simulink model "Landing_VV"  (R2018b)
settings: Solver=ode4  StartTime=0.0  StopTime=simTime  FixedStep=dt  RelTol=1e-3
InitFcn:
  | SimulationInitialization
StopFcn:
  | SimulationEnd
values from neighbouring files (symbols this model uses):
  Alt = 1000 + TerrainHeight    [SimulationStateConfig.m]
  C = GeneticOpt.C    [SimulationCostFunction.m]
  CartRange_m = MaxAftCartLocX_m - MaxFwdCartLocX_m    (= 1.8505)    [SimulationWSMConfig.m]
  DP_init = 0.5*1.225*V_init^2    [SimulationControlConfig16P.m]    (also in SimulationControlConfig16P_F0.m; SimulationControlConfig16P_F2.m; SimulationControlConfig16P_LEGACY.m; SimulationControlConfigTAILLESS.m)
  dt = DLLSim.dt    [SimulationTimeStep.m]    (also in SimulationTrim.m = 0.02)
  ElevatorMax = 25    [SimulationControlConfig16P.m]    (also in SimulationControlConfig16P_F0.m; SimulationControlConfig16P_F2.m; SimulationControlConfig16P_LEGACY.m; SimulationControlConfigTAILLESS.m)
  EngineLhFuelCut = 0    [SimulationAircraftConfig.m]
  EngineRhFuelCut = 0    [SimulationAircraftConfig.m]
  ftvStaticPositionError = 1/1.18    (= 0.847457627119)    [SimulationSensorConfig16P.m]    (also in SimulationSensorConfig16P_LEGACY.m; SimulationSensorConfigTAILLESS7P.m = 1; SimulationSensorConfigUTAIL7P.m = 1)
  g = 9.81    [SimulationStateConfig.m]
  GustSpd_Kts = testPlans(testIndx).gustSpd    [SimulationStateConfig.m]
  GustTriggerVal = testPlans(testIndx).gustTriggerVal    [SimulationStateConfig.m]
  m = 13.1784    [InertiaEstimatorBWB.m]    (also in SimulationControlConfig16P.m = MassBWB; SimulationControlConfig16P_F0.m = MassBWB; SimulationControlConfig16P_F2.m = MassBWB; SimulationControlConfig16P_LEGACY.m = MassBWB)
  MaxAftCartLocX_m = 2.5327    [SimulationWSMConfig.m]
  MaxFwdCartLocX_m = 0.6822    [SimulationWSMConfig.m]
  nMax_User = 2.6    [SimulationControlConfig16P.m]    (also in SimulationControlConfig16P_F0.m; SimulationControlConfig16P_F2.m; SimulationControlConfig16P_LEGACY.m; SimulationControlConfigTAILLESS.m = 2.5)
  nMin_User = -1.3    [SimulationControlConfig16P.m]    (also in SimulationControlConfig16P_F0.m; SimulationControlConfig16P_F2.m; SimulationControlConfig16P_LEGACY.m; SimulationControlConfigTAILLESS.m = -1)
  SimObj = CompiledSimulink(DLL_Name)    [SimulationTrim.m]
  taxiTrackOffset = testPlans(testIndx).rolloutTrackOffset    [SimulationControlConfig16P.m]    (also in SimulationControlConfig16P_F0.m; SimulationControlConfig16P_F2.m; SimulationControlConfig16P_LEGACY.m; SimulationControlConfigTAILLESS.m)
  V_init = Speed*0.5144    [SimulationControlConfig16P.m]    (also in SimulationControlConfig16P_F0.m; SimulationControlConfig16P_F2.m; SimulationControlConfig16P_LEGACY.m; SimulationControlConfigTAILLESS.m)
  WindDir_Deg = testPlans(testIndx).winds(3)    [SimulationStateConfig.m]
  WindSpd_Kts = testPlans(testIndx).winds(1)    [SimulationStateConfig.m]
  WindVertSpd_Kts = 0    [SimulationStateConfig.m]
  WOWarmed = 1    [SimulationControlConfig16P.m]    (also in SimulationControlConfig16P_F0.m; SimulationControlConfig16P_F2.m; SimulationControlConfig16P_LEGACY.m; SimulationControlConfigTAILLESS.m)
undefined symbols (not defined in the file or in its folder): DiscIntNeverNeededParam, DLLSim, DLLSimStep, sigbuilder_block, Trim_piccoloInCmd, Trim_REFSI_FD_IN_nmodeCgShifterCmd_Flag, Trim_REFSI_FD_IN_nmodeCgShifterCmd_Ft, Trim_REFSI_FD_IN_nmodeCgShifterNRCActive, WSMCart
libraries: Lib_Piccolo x16, simulink x10, aerolibatmos2 x2, Lib_HStab x1
(part 1 of 3)
settings Model: Creator=JSheng  LastModifiedBy=JCdFFigueira

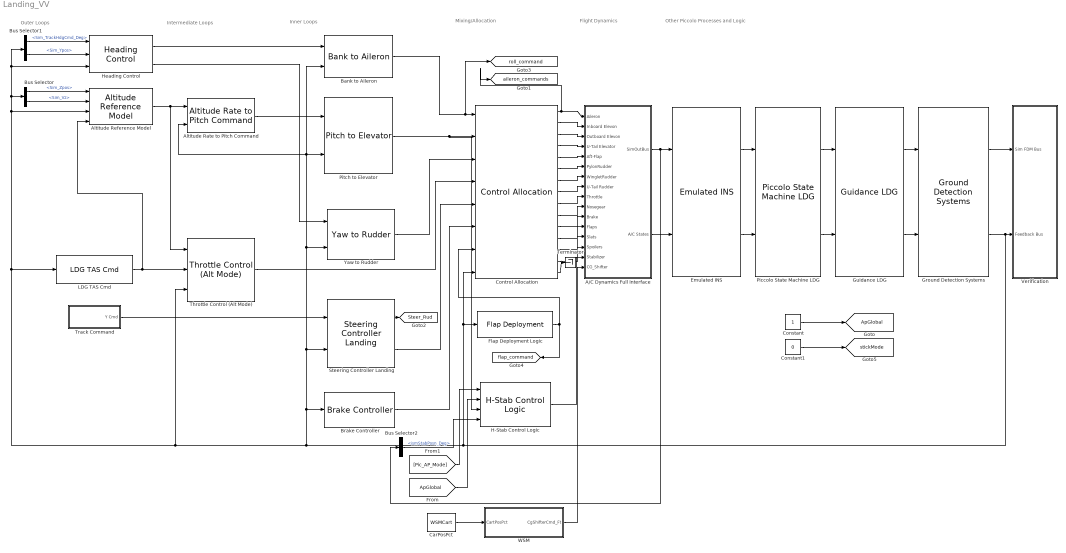
== system Landing_VV ==
  note: Outer Loops
  note: Intermediate Loops
  note: Inner Loops
  note: Flight Dynamics
  note: Other Piccolo Processes and Logic
  note: Mixing/Allocation
  A/C Dynamics Full Interface : Subsystem  AncestorBlock=Lib_Piccolo/A//C Dynamics Full Interface
  Altitude Rate to Pitch Command : Lib_Piccolo/Altitude Rate to Pitch Command  SystemSampleTime=-1
  Altitude Reference Model : Lib_Piccolo/Altitude Reference Model  SystemSampleTime=-1
  Bank to Aileron : Lib_Piccolo/Bank to Aileron  SystemSampleTime=-1
  Brake Controller : Lib_Piccolo/Brake Controller  SystemSampleTime=-1
  Bus Selector : BusSelector  OutputSignals=Sim_Zpos,Sim_Vz
  Bus Selector1 : BusSelector  OutputSignals=Sim_TrackHdgCmd_Deg,Sim_Ypos
  Bus Selector2 : BusSelector  OutputSignals=ismStabPosn_Deg
  CarPosPct : Constant  Value=WSMCart
  Constant : Constant
  Constant1 : Constant  Value=0
  Control Allocation : Lib_Piccolo/Control Allocation  SystemSampleTime=-1
  Emulated INS : Lib_Piccolo/Emulated INS  SystemSampleTime=-1
  Flap Deployment Logic : Lib_Piccolo/Flap Deployment  SystemSampleTime=-1
  Ground Detection Systems : Lib_Piccolo/Ground Detection Systems  SystemSampleTime=-1
  Guidance LDG : Lib_Piccolo/Guidance LDG  SystemSampleTime=-1
  H-Stab Control Logic : Lib_HStab/H-Stab Control Logic  SystemSampleTime=-1  VariantControl=Variant1  LabelModeActiveChoice=FTV == 4
  Heading Control : Lib_Piccolo/Heading Control  SystemSampleTime=-1
  LDG TAS Cmd : Lib_Piccolo/LDG TAS Cmd  SystemSampleTime=-1
  Piccolo State Machine LDG : Lib_Piccolo/Piccolo State Machine LDG  SystemSampleTime=-1
  Pitch to Elevator : Lib_Piccolo/Pitch to Elevator  SystemSampleTime=-1
  Steering Controller Landing : Lib_Piccolo/Steering Controller Landing  SystemSampleTime=-1
  Terminator : Terminator
  Throttle Control (Alt Mode) : Lib_Piccolo/Throttle Control (Alt Mode)  SystemSampleTime=-1
  Track Command : Subsystem
  Verification : Subsystem
  WSM : Subsystem
  Yaw to Rudder : Lib_Piccolo/Yaw to Rudder  SystemSampleTime=-1
  tag scope: ApGlobal=global, Steer_Rud=global, aileron_commands=global, flap_command=global, roll_command=global, stickMode=global
  wires:
  Pitch to Elevator/1 -> H-Stab Control Logic/3, Control Allocation/2
  Altitude Rate to Pitch Command/1 -> Pitch to Elevator/1
  Bank to Aileron/1 -> [roll_command], Control Allocation/1
  Control Allocation/1 -> [aileron_commands], A/C Dynamics Full Interface/1(Aileron)
  Control Allocation/2 -> A/C Dynamics Full Interface/2(Inboard Elevon)
  Control Allocation/3 -> A/C Dynamics Full Interface/3(Outboard Elevon)
  Control Allocation/4 -> A/C Dynamics Full Interface/4(U-Tail Elevator)
  Control Allocation/5 -> A/C Dynamics Full Interface/5(Aft-Flap)
  Control Allocation/6 -> A/C Dynamics Full Interface/6("PylonRudder ")
  Control Allocation/7 -> A/C Dynamics Full Interface/7(WingletRudder)
  Control Allocation/8 -> A/C Dynamics Full Interface/8(U-Tail Rudder)
  Control Allocation/9 -> A/C Dynamics Full Interface/9("Throttle ")
  Throttle Control (Alt Mode)/1 -> Control Allocation/4
  Heading Control/1 -> Bank to Aileron/1
  A/C Dynamics Full Interface/2(A/C States) -> Emulated INS/2
  LDG TAS Cmd/1 -> Throttle Control (Alt Mode)/2, Altitude Reference Model/4
  A/C Dynamics Full Interface/1(SimOutBus) -> Bus Selector2/1, Emulated INS/1
  Control Allocation/10 -> A/C Dynamics Full Interface/10(Nosegear)
  Control Allocation/11 -> A/C Dynamics Full Interface/11(Brake)
  Track Command/1(Y Cmd) -> Steering Controller Landing/1
  Brake Controller/1 -> Control Allocation/6
  Steering Controller Landing/2 -> Control Allocation/5
  Steering Controller Landing/1 -> [Steer_Rud]
  Yaw to Rudder/1 -> Control Allocation/3
  Emulated INS/2 -> Piccolo State Machine LDG/2
  Emulated INS/1 -> Piccolo State Machine LDG/1
  Ground Detection Systems/2 -> Verification/2(Feedback Bus), LDG TAS Cmd/1, Bus Selector/1, Heading Control/3, Bus Selector1/1, Altitude Reference Model/3, Throttle Control (Alt Mode)/3, Brake Controller/1, Steering Controller Landing/2, Pitch to Elevator/2, Bank to Aileron/2, Altitude Rate to Pitch Command/2, Yaw to Rudder/2, Flap Deployment Logic/1, Control Allocation/8
  Ground Detection Systems/1 -> Verification/1(Sim FDM Bus)
  Piccolo State Machine LDG/2 -> Guidance LDG/2
  Guidance LDG/2 -> Ground Detection Systems/2
  Piccolo State Machine LDG/1 -> Guidance LDG/1
  Guidance LDG/1 -> Ground Detection Systems/1
  Altitude Reference Model/1 -> Throttle Control (Alt Mode)/1, Altitude Rate to Pitch Command/1
  Bus Selector/2 -> Altitude Reference Model/2  "<Sim_Vz>"
  Bus Selector/1 -> Altitude Reference Model/1  "<Sim_Zpos>"
  Bus Selector1/2 -> Heading Control/2  "<Sim_Ypos>"
  Heading Control/2 -> Yaw to Rudder/1
  Bus Selector1/1 -> Heading Control/1  "<Sim_TrackHdgCmd_Deg>"
  Control Allocation/12 -> A/C Dynamics Full Interface/12(Flaps)
  Control Allocation/13 -> A/C Dynamics Full Interface/13(Slats)
  Control Allocation/14 -> A/C Dynamics Full Interface/14(Spoilers)
  Constant/1 -> [ApGlobal]
  Control Allocation/15 -> Terminator/1
  Flap Deployment Logic/1 -> [flap_command], Control Allocation/7
  Constant1/1 -> [stickMode]
  H-Stab Control Logic/1 -> A/C Dynamics Full Interface/15(Stabilizer)
  [ApGlobal] -> H-Stab Control Logic/2
  [Pic_AP_Mode] -> H-Stab Control Logic/1
  Bus Selector2/1 -> H-Stab Control Logic/4  "<ismStabPosn_Deg>"
  WSM/1(CgShifterCmd_Ft) -> A/C Dynamics Full Interface/16(CG_Shifter)
  CarPosPct/1 -> WSM/1(CartPosPct)

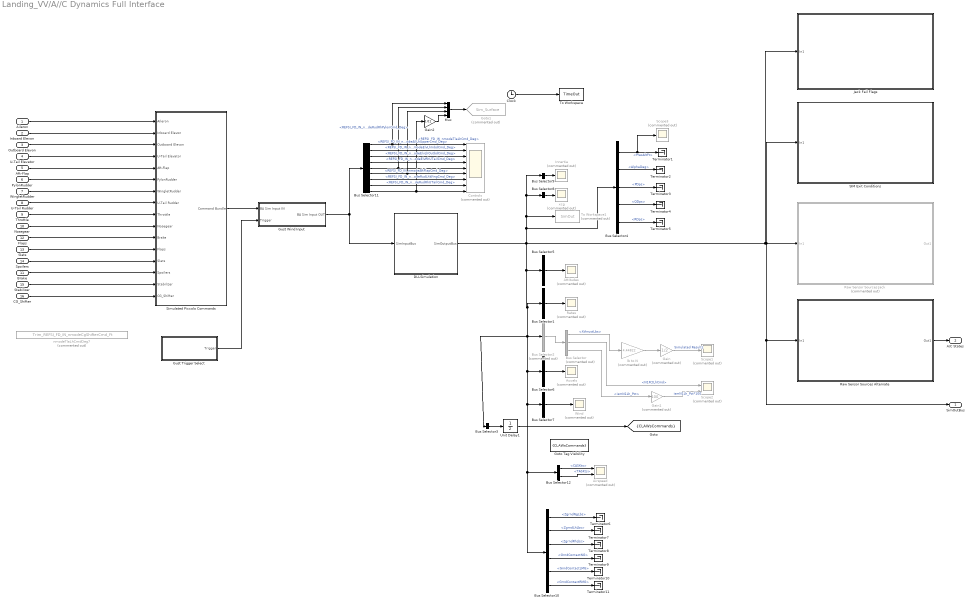
== system Landing_VV/A//C Dynamics Full Interface ==
  Aileron : Inport
  Inboard Elevon : Inport  Port=2
  Outboard Elevon : Inport  Port=3
  U-Tail Elevator : Inport  Port=4
  Aft-Flap : Inport  Port=5
  "PylonRudder " : Inport  Port=6
  WingletRudder : Inport  Port=7
  U-Tail Rudder : Inport  Port=8
  "Throttle " : Inport  Port=9
  Nosegear : Inport  Port=10
  Brake : Inport  Port=11
  Flaps : Inport  Port=12
  Slats : Inport  Port=13
  Spoilers : Inport  Port=14
  Stabilizer : Inport  Port=15
  CG_Shifter : Inport  Port=16
  Accels : Scope  Commented=on
  Airspeed : Scope  Commented=on  NumInputPorts=2
  Attitudes : Scope  Commented=on
  Bus Selector : BusSelector  Commented=on  OutputSignals=XthrustLbs,N1PctLhCmd,ismN1Lh_Pct
  Bus Selector1 : BusSelector  OutputSignals=PDps,QDps,RDps  OutputAsBus=on
  Bus Selector10 : BusSelector  OutputSignals=ZgrndNgLbs,ZgrndLhLbs,ZgrndRhLbs,GrndContactNG,GrndContactLMG,GrndContactRMG
  Bus Selector11 : BusSelector  OutputSignals=REFSI_FD_IN_nmodeAilLhUpperCmd_Deg,REFSI_FD_IN_nmodeElvLhInbdCmd_Deg,REFSI_FD_IN_nmodeElvLhOutbdCmd_Deg,REFSI_FD_IN_nmodeElvRhUTailCmd_Deg,REFSI_FD_IN_nmodeAftFlapCmd_Deg,REFSI_FD_IN_nmodeRudRhPylonCmd_Deg,REFSI_FD_IN_nmodeRudLhWingCmd_Deg,REFSI_FD_IN_nmodeRudRhUTailCmd_Deg,REFSI_FD_IN_nmodeTlaLhCmd_Deg
  Bus Selector12 : BusSelector  OutputSignals=CASKts,TASKts
  Bus Selector2 : BusSelector  Commented=on  OutputSignals=XthrustLbs,N1PctLhCmd,ismN1Lh_Pct,ismFuelBurnRateLh_Lpm,ismFuelBurntLh_Lbs  OutputAsBus=on
  Bus Selector3 : BusSelector  OutputSignals=REFSI_AC_OUT_nmodeRudLhWingCmd_Deg,REFSI_AC_OUT_nmodeAilLhLowerCmd_Deg,REFSI_AC_OUT_nmodeAilLhUpperCmd_Deg,REFSI_AC_OUT_nmodeElvLhOutbdCmd_Deg,REFSI_AC_OUT_nmodeElvLhInbdCmd_Deg,REFSI_AC_OUT_nmodeRudLhPylonCmd_Deg,REFSI_AC_OUT_nmodeRudLhUTailCmd_Deg,REFSI_AC_OUT_nmodeElvLhUTailCmd_Deg,REFSI_AC_OUT_nmodeAftFlapCmd_Deg,REFSI_AC_OUT_nmodeElvRhUTailCmd_Deg,REFSI_AC_OUT_nmodeRudRhUTailCmd_Deg,REFSI_AC_OUT_nmodeRudRhPylonCmd_Deg,REFSI_AC_OUT_nmodeElvRhInbdCmd_Deg,REFSI_AC_OUT_nmodeElvRhOutbdCmd_Deg,REFSI_AC_OUT_nmodeAilRhUpperCmd_Deg,REFSI_AC_OUT_nmodeAilRhLowerCmd_Deg,REFSI_AC_OUT_nmodeRudRhWingCmd_Deg  OutputAsBus=on
  Bus Selector4 : BusSelector  OutputSignals=PresAltFt,AlphaDeg,PDps,QDps,RDps
  Bus Selector5 : BusSelector  OutputSignals=PhiDeg,ThetaDeg,PsiDeg  OutputAsBus=on
  Bus Selector6 : BusSelector  OutputSignals=NxG,NyG,NzG  OutputAsBus=on
  Bus Selector7 : BusSelector  OutputSignals=WindUFtps,WindVFtps,WindWFtps  OutputAsBus=on
  Bus Selector8 : BusSelector  OutputSignals=XcgPctMAC  OutputAsBus=on
  Bus Selector9 : BusSelector  OutputSignals=IxxLbsInch2,IyyLbsInch2,IzzLbsInch2,IxzLbsInch2  OutputAsBus=on
  Clock : Clock
  Controls : Scope  Commented=on  NumInputPorts=9
  DLLSimulation : Subsystem
  Gain : Gain  Commented=on  Gain=1/2
  Gain1 : Gain  Commented=on  Gain=100
  Gain2 : Gain  Gain=0.01
  Goto Tag Visibility : GotoTagVisibility  GotoTag=CLAWsCommands
  Goto1 : Goto  Commented=on  GotoTag=Sim_Surface  TagVisibility=global
  Gust Trigger Select : Subsystem  Variant=on
  Gust Wind Input : Subsystem  Variant=on
  Innertia : Scope  Commented=on
  Jack Fail Flags : Subsystem
  Mux : Mux
  Rates : Scope  Commented=on
  Raw Sensor Sources Alternate : Subsystem
  Raw Sensor Sources Jack : Subsystem  Commented=on
  SIM Exit Conditions : Subsystem
  Scope1 : Scope  Commented=on
  Scope2 : Scope  Commented=on  NumInputPorts=2
  Scope3 : Scope  Commented=on
  Simulated Piccolo Commands : Subsystem  Variant=on
  Terminator{1..11} (11 alike) : Terminator
  To Workspace : ToWorkspace  VariableName=TimeOut  SaveFormat=Structure With Time  SampleTime=-1
  To Workspace1 : ToWorkspace  Commented=on  VariableName=SimOut  SaveFormat=Timeseries  SampleTime=-1
  Unit Delay1 : UnitDelay  SampleTime=-1
  Wind : Scope  Commented=on
  lb to N : Gain  Commented=on  Gain=4.44822
  nmodeTlaLhCmdDeg7 : Constant  Commented=on  Value=Trim_REFSI_FD_IN_nmodeCgShifterCmd_Ft
  xcg : Scope  Commented=on
  SimOutBus : Outport
  A/C States : Outport  Port=2
  tag scope: CLAWsCommands=scoped
  wires:
  "Throttle "/1 -> Simulated Piccolo Commands/9("Throttle ")
  Outboard Elevon/1 -> Simulated Piccolo Commands/3(Outboard Elevon)
  Nosegear/1 -> Simulated Piccolo Commands/10(Nosegear)
  Spoilers/1 -> Simulated Piccolo Commands/13(Slats)
  Gust Trigger Select/1(Trigger) -> Gust Wind Input/2(Trigger)
  Slats/1 -> Simulated Piccolo Commands/12(Flaps)
  Flaps/1 -> Simulated Piccolo Commands/11(Brake)
  Stabilizer/1 -> Simulated Piccolo Commands/15(Stabilizer)
  Inboard Elevon/1 -> Simulated Piccolo Commands/2(Inboard Elevon)
  U-Tail Elevator/1 -> Simulated Piccolo Commands/4(U-Tail Elevator)
  U-Tail Rudder/1 -> Simulated Piccolo Commands/8(U-Tail Rudder)
  Simulated Piccolo Commands/1(Command Bundle) -> Gust Wind Input/1(BA Sim Input IN)
  "PylonRudder "/1 -> Simulated Piccolo Commands/6("PylonRudder ")
  Brake/1 -> Simulated Piccolo Commands/14(Spoilers)
  WingletRudder/1 -> Simulated Piccolo Commands/7(WingletRudder)
  Aft-Flap/1 -> Simulated Piccolo Commands/5(Aft-Flap)
  Aileron/1 -> Simulated Piccolo Commands/1(Aileron)
  Raw Sensor Sources Alternate/1(Out1) -> A/C States/1
  DLLSimulation/1(SimOutputBus) -> To Workspace1/1, Bus Selector8/1, Bus Selector9/1, Bus Selector4/1, Bus Selector1/1, Bus Selector2/1, Bus Selector3/1, Bus Selector6/1, Bus Selector7/1, Bus Selector12/1, Bus Selector10/1, Bus Selector5/1, Raw Sensor Sources Jack/1(In1), SimOutBus/1, Raw Sensor Sources Alternate/1(In1), SIM Exit Conditions/1(In1), Jack Fail Flags/1(In1)
  Bus Selector10/6 -> Terminator11/1  "<GrndContactRMG>"
  Bus Selector10/5 -> Terminator10/1  "<GrndContactLMG>"
  Bus Selector10/4 -> Terminator9/1  "<GrndContactNG>"
  Bus Selector10/3 -> Terminator8/1  "<ZgrndRhLbs>"
  Bus Selector10/2 -> Terminator7/1  "<ZgrndLhLbs>"
  Bus Selector10/1 -> Terminator6/1  "<ZgrndNgLbs>"
  Gain2/1 -> Mux/4
  Mux/1 -> Goto1/1
  Bus Selector11/9 -> Controls/9, Gain2/1  "<REFSI_FD_IN_nmodeTlaLhCmd_Deg>"
  Bus Selector11/8 -> Controls/8  "<REFSI_FD_IN_nmodeRudRhUTailCmd_Deg>"
  Bus Selector11/7 -> Controls/7  "<REFSI_FD_IN_nmodeRudLhWingCmd_Deg>"
  Bus Selector11/6 -> Mux/3, Controls/6  "<REFSI_FD_IN_nmodeRudRhPylonCmd_Deg>"
  Bus Selector11/5 -> Mux/2, Controls/5  "<REFSI_FD_IN_nmodeAftFlapCmd_Deg>"
  Bus Selector11/4 -> Controls/4  "<REFSI_FD_IN_nmodeElvRhUTailCmd_Deg>"
  Bus Selector11/3 -> Controls/3  "<REFSI_FD_IN_nmodeElvLhOutbdCmd_Deg>"
  Bus Selector11/2 -> Controls/2  "<REFSI_FD_IN_nmodeElvLhInbdCmd_Deg>"
  Bus Selector11/1 -> Controls/1, Mux/1  "<REFSI_FD_IN_nmodeAilLhUpperCmd_Deg>"
  Bus Selector1/1 -> Rates/1
  Bus Selector12/1 -> Airspeed/1  "<CASKts>"
  Bus Selector4/4 -> Terminator4/1  "<QDps>"
  Gain1/1 -> Scope2/2  "ismN1Lh_Pct*100"
  Bus Selector4/2 -> Terminator2/1  "<AlphaDeg>"
  Bus Selector4/3 -> Terminator3/1  "<PDps>"
  Bus Selector5/1 -> Attitudes/1
  Unit Delay1/1 -> [CLAWsCommands]
  Bus Selector12/2 -> Airspeed/2  "<TASKts>"
  Bus Selector9/1 -> Innertia/1
  Bus Selector3/1 -> Unit Delay1/1
  Bus Selector6/1 -> Accels/1
  Bus Selector8/1 -> xcg/1
  Bus Selector4/5 -> Terminator5/1  "<RDps>"
  Gain/1 -> Scope1/1  "Simulated Results"
  Bus Selector/3 -> Gain1/1  "<ismN1Lh_Pct>"
  Bus Selector/1 -> lb to N/1  "<XthrustLbs>"
  lb to N/1 -> Gain/1
  Bus Selector/2 -> Scope2/1  "<N1PctLhCmd>"
  Bus Selector4/1 -> Terminator1/1, Scope3/1  "<PresAltFt>"
  Clock/1 -> To Workspace/1
  Bus Selector7/1 -> Wind/1
  Bus Selector2/1 -> Bus Selector/1
  Gust Wind Input/1(BA Sim Input OUT) -> DLLSimulation/1(SimInputBus), Bus Selector11/1
  CG_Shifter/1 -> Simulated Piccolo Commands/16(CG_Shifter)

== system Landing_VV/Track Command ==
  In-Flight Cmd : Constant  Value=taxiTrackOffset
  Switch : Switch  Threshold=11
  Taxi Cmd : Constant  Value=taxiTrackOffset
  Y Cmd : Outport
  wires:
  [Pic_AP_Mode] -> Switch/2
  Switch/1 -> Y Cmd/1
  Taxi Cmd/1 -> Switch/1
  In-Flight Cmd/1 -> Switch/3

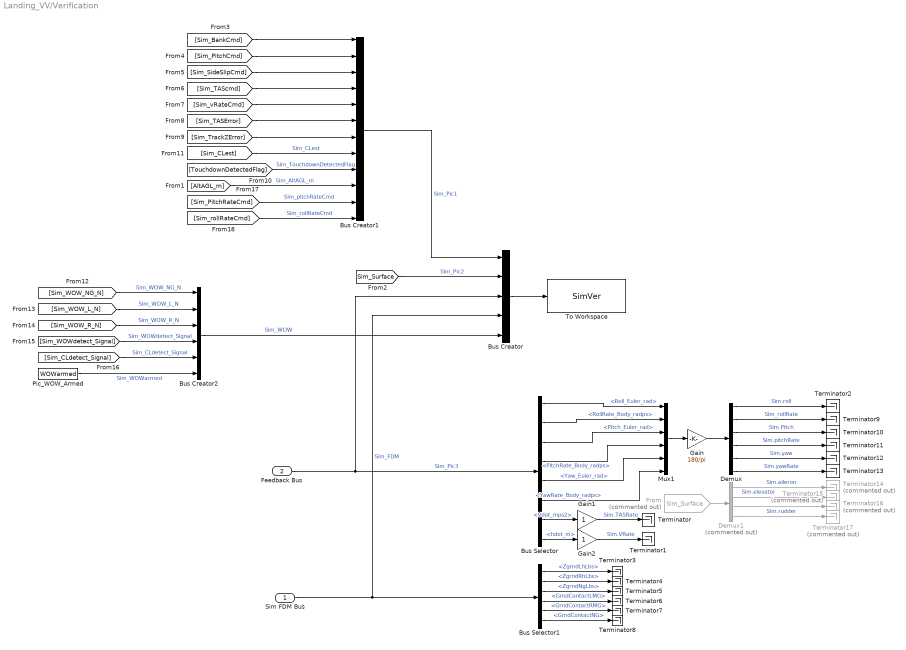
== system Landing_VV/Verification ==
  Sim FDM Bus : Inport
  Feedback Bus : Inport  Port=2
  Bus Creator : BusCreator  Inputs=5
  Bus Creator1 : BusCreator  Inputs=12
  Bus Creator2 : BusCreator  Inputs=6
  Bus Selector : BusSelector  OutputSignals=Roll_Euler_rad,RollRate_Body_radps,Pitch_Euler_rad,PitchRate_Body_radps,Yaw_Euler_rad,YawRate_Body_radps,Vdot_mps2,hdot_m
  Bus Selector1 : BusSelector  OutputSignals=ZgrndLhLbs,ZgrndRhLbs,ZgrndNgLbs,GrndContactLMG,GrndContactRMG,GrndContactNG
  Demux : Demux  Outputs=6
  Demux1 : Demux  Commented=on
  From : From  Commented=on  GotoTag=Sim_Surface  TagVisibility=global
  Gain : Gain  Gain=180/pi
  Gain1 : Gain
  Gain2 : Gain
  Mux1 : Mux  Inputs=6
  Pic_WOW_Armed : Constant  Value=WOWarmed
  Terminator{,1..13} (14 alike) : Terminator
  Terminator{14..17} (4 alike) : Terminator  Commented=on
  To Workspace : ToWorkspace  VariableName=SimVer  SaveFormat=Timeseries  SampleTime=-1
  wires:
  Bus Selector1/4 -> Terminator6/1  "<GrndContactLMG>"
  Bus Selector/3 -> Mux1/3  "<Pitch_Euler_rad>"
  Bus Selector/2 -> Mux1/2  "<RollRate_Body_radps>"
  Mux1/1 -> Gain/1
  Bus Selector/7 -> Gain1/1  "<Vdot_mps2>"
  Bus Selector/6 -> Mux1/6  "<YawRate_Body_radps>"
  Bus Selector/5 -> Mux1/5  "<Yaw_Euler_rad>"
  Bus Selector/4 -> Mux1/4  "<PitchRate_Body_radps>"
  Bus Selector1/5 -> Terminator7/1  "<GrndContactRMG>"
  Bus Selector1/3 -> Terminator5/1  "<ZgrndNgLbs>"
  Bus Selector/1 -> Mux1/1  "<Roll_Euler_rad>"
  Feedback Bus/1 -> Bus Creator/3, Bus Selector/1  "Sim_Pic3"
  Gain/1 -> Demux/1
  Bus Selector1/1 -> Terminator3/1  "<ZgrndLhLbs>"
  Bus Selector1/6 -> Terminator8/1  "<GrndContactNG>"
  Bus Selector1/2 -> Terminator4/1  "<ZgrndRhLbs>"
  Bus Selector/8 -> Gain2/1  "<hdot_m>"
  Sim FDM Bus/1 -> Bus Creator/4, Bus Selector1/1  "Sim_FDM"
  From/1 -> Demux1/1
  Gain2/1 -> Terminator1/1  "Sim.VRate"
  Gain1/1 -> Terminator/1  "Sim.TASRate"
  Demux/1 -> Terminator2/1  "Sim.roll"
  Demux/2 -> Terminator9/1  "Sim_rollRate"
  Demux/3 -> Terminator10/1  "Sim.Pitch"
  Demux/4 -> Terminator11/1  "Sim.pitchRate"
  Demux/5 -> Terminator12/1  "Sim.yaw"
  Demux/6 -> Terminator13/1  "Sim.yawRate"
  Demux1/1 -> Terminator14/1  "Sim.aileron"
  Demux1/2 -> Terminator15/1  "Sim.elevator"
  Demux1/3 -> Terminator16/1  "Sim.rudder"
  Demux1/4 -> Terminator17/1
  Bus Creator/1 -> To Workspace/1
  [AltAGL_m] -> Bus Creator1/10  "Sim_AltAGL_m"
  [Sim_Surface] -> Bus Creator/2  "Sim_Pic2"
  [Sim_BankCmd] -> Bus Creator1/1
  [Sim_PitchCmd] -> Bus Creator1/2
  [Sim_SideSlipCmd] -> Bus Creator1/3
  [Sim_TAScmd] -> Bus Creator1/4
  [Sim_vRateCmd] -> Bus Creator1/5
  [Sim_TASError] -> Bus Creator1/6
  [Sim_TrackZError] -> Bus Creator1/7
  Bus Creator1/1 -> Bus Creator/1  "Sim_Pic1"
  [TouchdownDetectedFlag] -> Bus Creator1/9  "Sim_TouchdownDetectedFlag"
  [Sim_CLest] -> Bus Creator1/8  "Sim_CLest"
  [Sim_WOW_NG_N] -> Bus Creator2/1  "Sim_WOW_NG_N"
  [Sim_WOW_L_N] -> Bus Creator2/2  "Sim_WOW_L_N"
  [Sim_WOW_R_N] -> Bus Creator2/3  "Sim_WOW_R_N"
  [Sim_WOWdetect_Signal] -> Bus Creator2/4  "Sim_WOWdetect_Signal"
  Bus Creator2/1 -> Bus Creator/5  "Sim_WOW"
  Pic_WOW_Armed/1 -> Bus Creator2/6  "Sim_WOWarmed"
  [Sim_CLdetect_Signal] -> Bus Creator2/5  "Sim_CLdetect_Signal"
  [Sim_PitchRateCmd] -> Bus Creator1/11  "Sim_pitchRateCmd"
  [Sim_rollRateCmd] -> Bus Creator1/12  "Sim_rollRateCmd"

== system Landing_VV/WSM ==
  CartPosPct : Inport
  Constant : Constant  Value=MaxFwdCartLocX_m
  Gain : Gain  Gain=1/100
  Gain1 : Gain  Gain=CartRange_m
  Saturation : Saturate  UpperLimit=MaxAftCartLocX_m  LowerLimit=MaxFwdCartLocX_m
  Sum : Sum  Inputs=|++
  m2ft : Gain  Gain=3.280839895
  nmodeTlaLhCmdDeg7 : Constant  Commented=on  Value=Trim_REFSI_FD_IN_nmodeCgShifterCmd_Ft
  CgShifterCmd_Ft : Outport
  wires:
  CartPosPct/1 -> Gain/1
  Gain/1 -> Gain1/1
  Gain1/1 -> Sum/1
  Constant/1 -> Sum/2
  Sum/1 -> Saturation/1
  Saturation/1 -> m2ft/1
  m2ft/1 -> CgShifterCmd_Ft/1

== system Landing_VV/A//C Dynamics Full Interface/DLLSimulation ==
  SimInputBus : Inport
  Bus to Vector : BusToVector
  Bus2Vect2 : Subsystem  Commented=on
      mask init:
      | CurrentSys = gcs;
      | blockName = get_param(gcb,'Name');
      | 
      | CurBlk = [CurrentSys,'/',blockName];%Current block
      | BusSel = [CurrentSys,'/',blockName,'/BusSelector'];%BusSelectorBlock
      | BusMux = [CurrentSys,'/',blockName,'/Mux'];%Mux bloxk
      | 
      | 
      | 
      | Inputs = get_param(BusSel,'InputSignals');
      | 
      | 
      | outsig='';
      | for i=1:length(Inputs)
      |     outsig=[outsig Inputs{i} ','];
      | end;
      | outsig=outsig(1:length(outsig)-1);
      | 
      |     for nnn = 1:str2double(get_param(BusMux,'Inputs'))
      |         delete_line([CurrentSys '/' blockName],['BusSelector/' num2str(nnn)],['Mux/' num2str(nnn)])
      |     end
      |     
      | set_param(BusSel,'OutputSignals',outsig);
      | set_param(BusMux,'Inputs',num2str(length(Inputs)))
      | 
      | 
      | 
      |     
      |     for nnn = 1:length(Inputs)
      |         add_line([CurrentSys '/' blockName],['BusSelector/' num2str(nnn)],['Mux/' num2str(nnn)])
      |     end
  DLLSimulationStep : MATLABFcn  MATLABFcn=DLLSimStep(u,DLLSim.nDT)  OutputDimensions=DLLSim.nOuputs  SampleTime=dt
  Vector to Bus : Subsystem  Commented=on  mask{Nsigs=DLLSim.nOuputs}
      mask prompts: Nsigs "Signal Length"
  Vector to Bus v16_ : Subsystem  Variant=on
  SimOutputBus : Outport
  wires:
  SimInputBus/1 -> Bus to Vector/1
  Vector to Bus v16_/1(Out1) -> SimOutputBus/1
  DLLSimulationStep/1 -> Vector to Bus v16_/1(In1)
  Bus to Vector/1 -> DLLSimulationStep/1

== system Landing_VV/A//C Dynamics Full Interface/Gust Trigger Select ==
  note: 1) Add Subsystem or Model blocks as valid variant choices.
      | 2) You cannot connect blocks at this level. At simulation, connectivity is automatically
      | determined, based on the active variant and port name matching.
  Above AGL : Subsystem  VariantControl="GustTrigger == \"Above_AGL\""
  Above IAS : Subsystem  VariantControl="GustTrigger == \"Above_IAS\""
  Below AGL : Subsystem  VariantControl="GustTrigger == \"Below_AGL\""
  Trigger : Outport

== system Landing_VV/A//C Dynamics Full Interface/Gust Wind Input ==
  BA Sim Input IN : Inport
  Trigger : Inport  Port=2
  Gust Wind Model : Subsystem  VariantControl="GustType ~= \"NONE\""
  No Gust : Subsystem  VariantControl="GustType == \"NONE\""
  BA Sim Input OUT : Outport

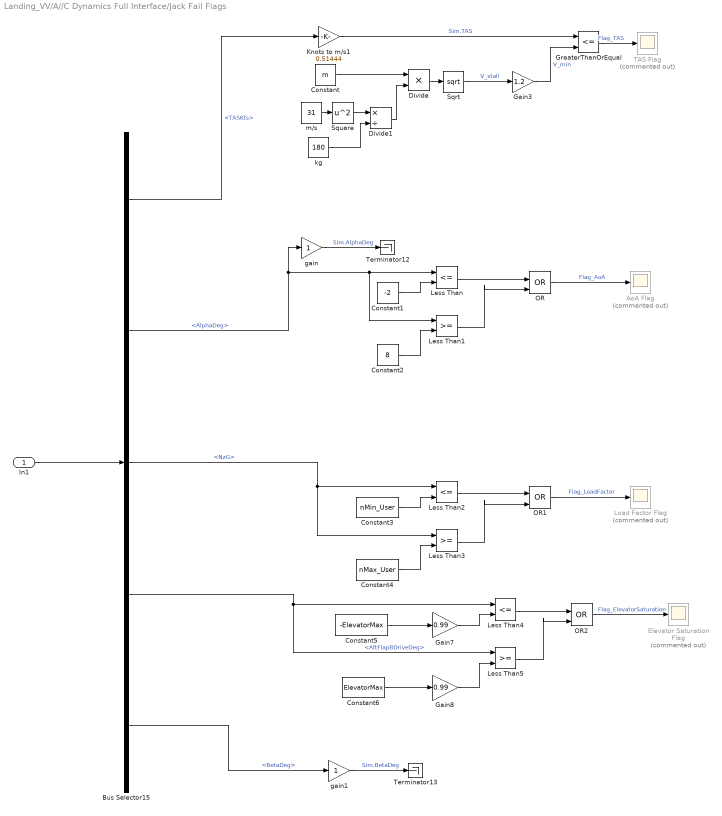
== system Landing_VV/A//C Dynamics Full Interface/Jack Fail Flags ==
  In1 : Inport
  AoA Flag : Scope  Commented=on
  Bus Selector15 : BusSelector  OutputSignals=TASKts,AlphaDeg,NzG,AftFlapBDriveDeg,BetaDeg
  Constant : Constant  Value=m
  Constant1 : Constant  Value=-2
  Constant2 : Constant  Value=8
  Constant3 : Constant  Value=nMin_User
  Constant4 : Constant  Value=nMax_User
  Constant5 : Constant  Value=-ElevatorMax
  Constant6 : Constant  Value=ElevatorMax
  Divide : Product  Inputs=**
  Divide1 : Product  Inputs=*/
  Elevator Saturation Flag : Scope  Commented=on
  Gain3 : Gain  Gain=1.2
  Gain7 : Gain  Gain=0.99
  Gain8 : Gain  Gain=0.99
  GreaterThanOrEqual : RelationalOperator  Operator=<=  OutDataTypeStr=boolean  RndMeth=Simplest
  Knots to m/s1 : Gain  Gain=0.51444
  Less Than : RelationalOperator  Operator=<=  OutDataTypeStr=boolean  RndMeth=Simplest
  Less Than1 : RelationalOperator  OutDataTypeStr=boolean  RndMeth=Simplest
  Less Than2 : RelationalOperator  Operator=<=  OutDataTypeStr=boolean  RndMeth=Simplest
  Less Than3 : RelationalOperator  OutDataTypeStr=boolean  RndMeth=Simplest
  Less Than4 : RelationalOperator  Operator=<=  OutDataTypeStr=boolean  RndMeth=Simplest
  Less Than5 : RelationalOperator  OutDataTypeStr=boolean  RndMeth=Simplest
  "Load Factor Flag " : Scope  Commented=on
  OR : Logic  Operator=OR  IconShape=distinctive  AllPortsSameDT=off  OutDataTypeStr=boolean
  OR1 : Logic  Operator=OR  IconShape=distinctive  AllPortsSameDT=off  OutDataTypeStr=boolean
  OR2 : Logic  Operator=OR  IconShape=distinctive  AllPortsSameDT=off  OutDataTypeStr=boolean
  Sqrt : Sqrt  SaturateOnIntegerOverflow=on
  Square : Math  Operator=square  SaturateOnIntegerOverflow=on
  TAS Flag : Scope  Commented=on
  Terminator12 : Terminator
  Terminator13 : Terminator
  gain : Gain
  gain1 : Gain
  kg : Constant  Value=180
  m/s : Constant  Value=31
  wires:
  In1/1 -> Bus Selector15/1
  Constant3/1 -> Less Than2/2
  gain1/1 -> Terminator13/1  "Sim.BetaDeg"
  gain/1 -> Terminator12/1  "Sim.AlphaDeg"
  Constant5/1 -> Gain7/1
  Divide/1 -> Sqrt/1
  OR/1 -> AoA Flag/1  "Flag_AoA"
  Sqrt/1 -> Gain3/1  "V_stall"
  kg/1 -> Divide1/2
  OR1/1 -> "Load Factor Flag "/1  "Flag_LoadFactor"
  Square/1 -> Divide1/1
  Bus Selector15/5 -> gain1/1  "<BetaDeg>"
  GreaterThanOrEqual/1 -> TAS Flag/1  "Flag_TAS"
  Gain3/1 -> GreaterThanOrEqual/2  "V_min"
  Less Than1/1 -> OR/2
  Less Than3/1 -> OR1/2
  m/s/1 -> Square/1
  Bus Selector15/4 -> Less Than4/1, Less Than5/1  "<AftFlapBDriveDeg>"
  Knots to m/s1/1 -> GreaterThanOrEqual/1  "Sim.TAS"
  Constant/1 -> Divide/1
  Bus Selector15/1 -> Knots to m/s1/1  "<TASKts>"
  Less Than/1 -> OR/1
  Gain7/1 -> Less Than4/2
  Constant1/1 -> Less Than/2
  Constant2/1 -> Less Than1/2
  Less Than2/1 -> OR1/1
  OR2/1 -> Elevator Saturation Flag/1  "Flag_ElevatorSaturation"
  Less Than4/1 -> OR2/1
  Gain8/1 -> Less Than5/2
  Bus Selector15/2 -> Less Than/1, Less Than1/1, gain/1  "<AlphaDeg>"
  Bus Selector15/3 -> Less Than2/1, Less Than3/1  "<NzG>"
  Less Than5/1 -> OR2/2
  Constant4/1 -> Less Than3/2
  Constant6/1 -> Gain8/1
  Divide1/1 -> Divide/2

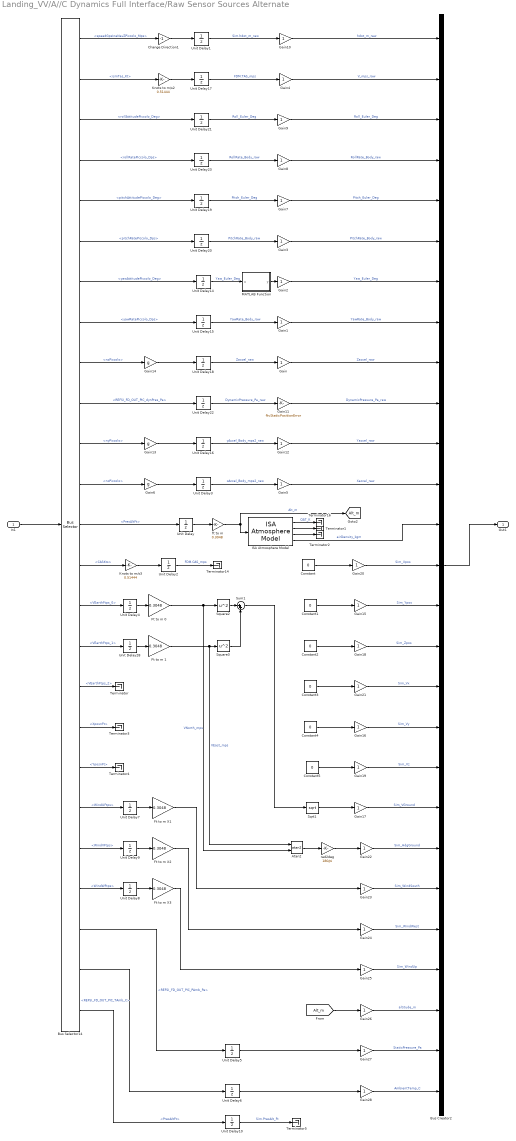
== system Landing_VV/A//C Dynamics Full Interface/Raw Sensor Sources Alternate ==
  In1 : Inport
  Atan2 : Trigonometry  Operator=atan2
  Bus Creator2 : BusCreator  Inputs=27
  Bus Selector14 : BusSelector  OutputSignals=speedGpsIneNavZPiccolo_Mps,ismTas_Kt,rollAttitudePiccolo_Deg,rollRatePiccolo_Dps,pitchAttitudePiccolo_Deg,pitchRatePiccolo_Dps,yawAttitudePiccolo_Deg,yawRatePiccolo_Dps,nzPiccolo,REFSI_FD_OUT_PIC_dynPres_Pa,nyPiccolo,nxPiccolo,PresAltFt,CASKts,VEarthFtps_0,VEarthFtps_1,VEarthFtps_2,XposnFt,YposnFt,WindUFtps,WindVFtps,WindWFtps,REFSI_FD_OUT_PIC_PAmb_Pa,REFSI_FD_OUT_PIC_TAmb_C,PresAltFt
  Change Direction1 : Gain  Gain=-1
  Constant{,1..5} (6 alike) : Constant  Value=0
  Ft to m 0 : Gain  Gain=0.3048
  Ft to m 1 : Gain  Gain=0.3048
  Ft to m X1 : Gain  Gain=0.3048
  Ft to m X2 : Gain  Gain=0.3048
  Ft to m X3 : Gain  Gain=0.3048
  Gain{,1..5,7..10,12,15..28} (25 alike) : Gain
  Gain11 : Gain  Gain=ftvStaticPositionError
  Gain13 : Gain  Gain=g
  Gain14 : Gain  Gain=g
  Gain6 : Gain  Gain=g
  ISA Atmosphere Model : aerolibatmos2/ISA Atmosphere Model  custom=off  g=9.80665  gamma=1.4  R=287.0531  L=0.0065  h_trop=11000  h_strat=20000  rho0=1.225  P0=101325  T0=288.15  h0=0
      settings: SourceProductName=Aerospace Blockset
  Knots to m/s2 : Gain  Gain=0.51444
  Knots to m/s3 : Gain  Gain=0.51444
  MATLAB Function : MATLAB Function  TreatAsAtomicUnit=on
  Sqrt1 : Sqrt  OutputSignalType=real  SaturateOnIntegerOverflow=on
  Square2 : Math  Operator=square  OutputSignalType=real  SaturateOnIntegerOverflow=on
  Square3 : Math  Operator=square  OutputSignalType=real  SaturateOnIntegerOverflow=on
  Sum1 : Sum  Inputs=|++
  Terminator{,1..5,14,16} (8 alike) : Terminator
  Unit Delay : UnitDelay  InitialCondition=Alt  SampleTime=dt
  Unit Delay{1,3..4,7..9,15..16,20,23,28} (11 alike) : UnitDelay  SampleTime=-1
  Unit Delay10 : UnitDelay  InitialCondition=10  SampleTime=-1
  Unit Delay14 : UnitDelay  InitialCondition=SimObj.Output.PsiDeg  SampleTime=-1
  Unit Delay17 : UnitDelay  InitialCondition=V_init  SampleTime=-1
  Unit Delay18 : UnitDelay  InitialCondition=g  SampleTime=-1
  Unit Delay19 : UnitDelay  InitialCondition=SimObj.Output.ThetaDeg  SampleTime=-1
  Unit Delay2 : UnitDelay  InitialCondition=V_init  SampleTime=dt
  Unit Delay21 : UnitDelay  InitialCondition=SimObj.Output.PhiDeg  SampleTime=-1
  Unit Delay22 : UnitDelay  InitialCondition=DP_init  SampleTime=-1
  Unit Delay5 : UnitDelay  InitialCondition=90000  SampleTime=-1
  Unit Delay6 : UnitDelay  InitialCondition=10  SampleTime=-1
  ft to m : Gain  Gain=0.3048
  rad2deg : Gain  Gain=180/pi
  Out1 : Outport
  tag scope: Alt_m=global
  wires:
  Unit Delay10/1 -> Terminator5/1  "Sim.PresAlt_Ft"
  Bus Selector14/25 -> Unit Delay10/1  "<PresAltFt>"
  Gain28/1 -> Bus Creator2/27  "AmbientTemp_C"
  Bus Selector14/24 -> Unit Delay6/1  "<REFSI_FD_OUT_PIC_TAmb_C>"
  Unit Delay6/1 -> Gain28/1
  Gain27/1 -> Bus Creator2/26  "StaticPressure_Pa"
  Unit Delay5/1 -> Gain27/1
  Bus Selector14/23 -> Unit Delay5/1  "<REFSI_FD_OUT_PIC_PAmb_Pa>"
  MATLAB Function/1(y) -> Gain2/1
  [Alt_m] -> Gain26/1
  Gain26/1 -> Bus Creator2/25  "altitude_m"
  Bus Selector14/19 -> Terminator4/1  "<YposnFt>"
  rad2deg/1 -> Gain22/1
  Atan2/1 -> rad2deg/1
  Unit Delay8/1 -> Ft to m X3/1
  Unit Delay9/1 -> Ft to m X2/1
  Unit Delay7/1 -> Ft to m X1/1
  Bus Selector14/22 -> Unit Delay8/1  "<WindWFtps>"
  Bus Selector14/21 -> Unit Delay9/1  "<WindVFtps>"
  Bus Selector14/20 -> Unit Delay7/1  "<WindUFtps>"
  Gain25/1 -> Bus Creator2/24  "Sim_WindUp"
  Ft to m X3/1 -> Gain25/1
  Ft to m X2/1 -> Gain24/1
  Ft to m X1/1 -> Gain23/1
  Sqrt1/1 -> Gain17/1
  Constant5/1 -> Gain19/1
  Constant4/1 -> Gain16/1
  Constant3/1 -> Gain21/1
  Constant2/1 -> Gain18/1
  Constant1/1 -> Gain15/1
  Constant/1 -> Gain20/1
  Gain24/1 -> Bus Creator2/23  "Sim_WindWest"
  Gain23/1 -> Bus Creator2/22  "Sim_WindSouth"
  Gain22/1 -> Bus Creator2/21  "Sim_HdgGround"
  Gain21/1 -> Bus Creator2/17  "Sim_Vx"
  Gain20/1 -> Bus Creator2/14  "Sim_Xpos"
  Gain19/1 -> Bus Creator2/19  "Sim_Vz"
  Gain18/1 -> Bus Creator2/16  "Sim_Zpos"
  Gain17/1 -> Bus Creator2/20  "Sim_VGround"
  Ft to m 1/1 -> Square3/1, Atan2/1  "VEast_mps"
  Square3/1 -> Sum1/2
  Ft to m 0/1 -> Square2/1, Atan2/2  "VNorth_mps"
  Square2/1 -> Sum1/1
  Sum1/1 -> Sqrt1/1
  Bus Selector14/18 -> Terminator3/1  "<XposnFt>"
  Gain16/1 -> Bus Creator2/18  "Sim_Vy"
  Gain15/1 -> Bus Creator2/15  "Sim_Ypos"
  Bus Selector14/17 -> Terminator/1  "<VEarthFtps_2>"
  Unit Delay4/1 -> Ft to m 0/1
  Unit Delay28/1 -> Ft to m 1/1
  Bus Selector14/16 -> Unit Delay28/1  "<VEarthFtps_1>"
  Bus Selector14/15 -> Unit Delay4/1  "<VEarthFtps_0>"
  Gain14/1 -> Unit Delay18/1
  Gain13/1 -> Unit Delay16/1
  Gain6/1 -> Unit Delay3/1
  Gain5/1 -> Bus Creator2/12  "Xaccel_raw"
  Unit Delay3/1 -> Gain5/1  "xAccel_Body_mps2_raw"
  Bus Selector14/12 -> Gain6/1  "<nxPiccolo>"
  Bus Selector14/11 -> Gain13/1  "<nyPiccolo>"
  Bus Selector14/10 -> Unit Delay22/1  "<REFSI_FD_OUT_PIC_dynPres_Pa>"
  Bus Selector14/9 -> Gain14/1  "<nzPiccolo>"
  Bus Selector14/8 -> Unit Delay15/1  "<yawRatePiccolo_Dps>"
  Bus Selector14/7 -> Unit Delay14/1  "<yawAttitudePiccolo_Deg>"
  Bus Selector14/6 -> Unit Delay20/1  "<pitchRatePiccolo_Dps>"
  Unit Delay1/1 -> Gain10/1  "Sim.hdot_m_raw"
  Bus Selector14/5 -> Unit Delay19/1  "<pitchAttitudePiccolo_Deg>"
  Bus Selector14/4 -> Unit Delay23/1  "<rollRatePiccolo_Dps>"
  Bus Selector14/3 -> Unit Delay21/1  "<rollAttitudePiccolo_Deg>"
  Bus Selector14/2 -> Knots to m/s2/1  "<ismTas_Kt>"
  Bus Selector14/1 -> Change Direction1/1  "<speedGpsIneNavZPiccolo_Mps>"
  Gain12/1 -> Bus Creator2/11  "Yaccel_raw"
  Gain11/1 -> Bus Creator2/10  "DynamicPressure_Pa_raw"
  Gain10/1 -> Bus Creator2/1  "hdot_m_raw"
  Gain9/1 -> Bus Creator2/3  "Roll_Euler_Deg"
  Gain8/1 -> Bus Creator2/4  "RollRate_Body_raw"
  Gain7/1 -> Bus Creator2/5  "Pitch_Euler_Deg"
  Gain3/1 -> Bus Creator2/6  "PitchRate_Body_raw"
  Gain2/1 -> Bus Creator2/7  "Yaw_Euler_Deg"
  Gain1/1 -> Bus Creator2/8  "YawRate_Body_raw"
  Gain/1 -> Bus Creator2/9  "Zaccel_raw"
  ISA Atmosphere Model/3 -> Terminator2/1
  ISA Atmosphere Model/2 -> Terminator1/1
  Bus Creator2/1 -> Out1/1
  Unit Delay21/1 -> Gain9/1  "Roll_Euler_Deg"
  Knots to m/s2/1 -> Unit Delay17/1
  ISA Atmosphere Model/4 -> Bus Creator2/13  "airDensity_kgm"
  Gain4/1 -> Bus Creator2/2  "V_mps_raw"
  In1/1 -> Bus Selector14/1
  Bus Selector14/14 -> Knots to m/s3/1  "<CASKts>"
  Unit Delay/1 -> ft to m/1
  Unit Delay15/1 -> Gain1/1  "YawRate_Body_raw"
  Unit Delay19/1 -> Gain7/1  "Pitch_Euler_Deg"
  Bus Selector14/13 -> Unit Delay/1  "<PresAltFt>"
  Unit Delay20/1 -> Gain3/1  "PitchRate_Body_raw"
  Unit Delay18/1 -> Gain/1  "Zaccel_raw"
  Unit Delay2/1 -> Terminator14/1  "FDM.CAS_mps"
  ft to m/1 -> [Alt_m], ISA Atmosphere Model/1  "Alt_m"
  Unit Delay14/1 -> MATLAB Function/1(u)  "Yaw_Euler_Deg"
  Unit Delay17/1 -> Gain4/1  "FDM.TAS_mps"
  Unit Delay16/1 -> Gain12/1  "yAccel_Body_mps2_raw"
  Unit Delay22/1 -> Gain11/1  "DynamicPressure_Pa_raw"
  ISA Atmosphere Model/1 -> Terminator16/1  "OAT_K"
  Unit Delay23/1 -> Gain8/1  "RollRate_Body_raw"
  Change Direction1/1 -> Unit Delay1/1
  Knots to m/s3/1 -> Unit Delay2/1

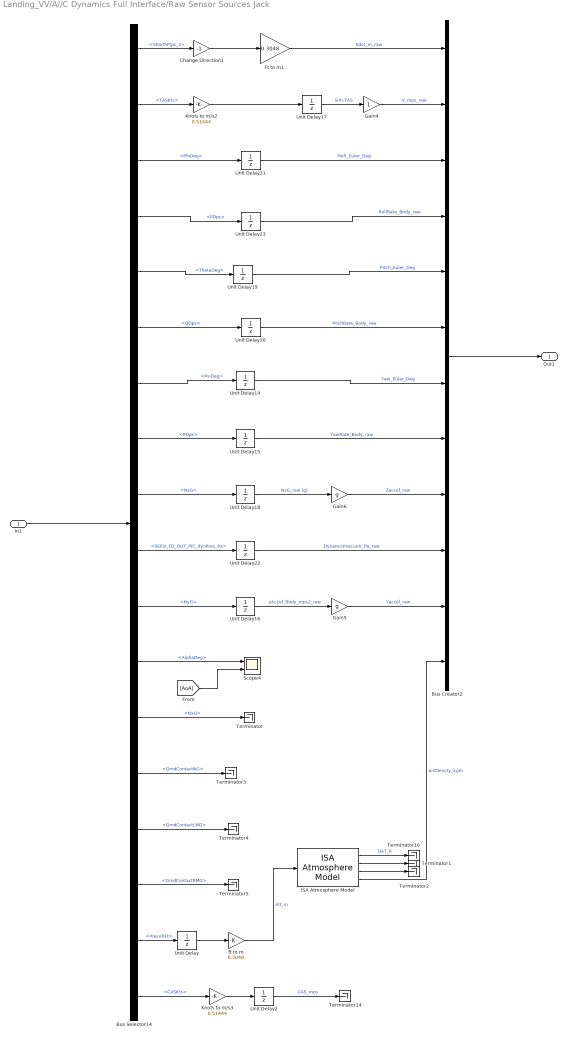
== system Landing_VV/A//C Dynamics Full Interface/Raw Sensor Sources Jack ==
  In1 : Inport
  Bus Creator2 : BusCreator  Inputs=12
  Bus Selector14 : BusSelector  OutputSignals=VEarthFtps_2,TASKts,PhiDeg,PDps,ThetaDeg,QDps,PsiDeg,RDps,NzG,REFSI_FD_OUT_PIC_dynPres_Pa,NyG,AlphaDeg,NxG,GrndContactNG,GrndContactLMG,GrndContactRMG,PresAltFt,CASKts
  Change Direction1 : Gain  Gain=-1
  Ft to m1 : Gain  Gain=0.3048
  Gain4 : Gain
  Gain5 : Gain  Gain=g
  Gain6 : Gain  Gain=g
  ISA Atmosphere Model : aerolibatmos2/ISA Atmosphere Model  custom=off  g=9.80665  gamma=1.4  R=287.0531  L=0.0065  h_trop=11000  h_strat=20000  rho0=1.225  P0=101325  T0=288.15  h0=0
      settings: SourceProductName=Aerospace Blockset
  Knots to m/s2 : Gain  Gain=0.51444
  Knots to m/s3 : Gain  Gain=0.51444
  Scope4 : Scope  NumInputPorts=2
  Terminator{,1..5,14,16} (8 alike) : Terminator
  Unit Delay : UnitDelay  InitialCondition=Alt  SampleTime=dt
  Unit Delay14 : UnitDelay  InitialCondition=SimObj.Output.PsiDeg  SampleTime=-1
  Unit Delay{15..16,20,23} (4 alike) : UnitDelay  SampleTime=-1
  Unit Delay17 : UnitDelay  InitialCondition=V_init  SampleTime=-1
  Unit Delay18 : UnitDelay  InitialCondition=1  SampleTime=-1
  Unit Delay19 : UnitDelay  InitialCondition=SimObj.Output.ThetaDeg  SampleTime=-1
  Unit Delay2 : UnitDelay  InitialCondition=V_init  SampleTime=dt
  Unit Delay21 : UnitDelay  InitialCondition=SimObj.Output.PhiDeg  SampleTime=-1
  Unit Delay22 : UnitDelay  InitialCondition=DP_init  SampleTime=-1
  ft to m : Gain  Gain=0.3048
  Out1 : Outport
  wires:
  Bus Selector14/14 -> Terminator3/1  "<GrndContactNG>"
  Bus Selector14/15 -> Terminator4/1  "<GrndContactLMG>"
  Bus Selector14/16 -> Terminator5/1  "<GrndContactRMG>"
  ISA Atmosphere Model/3 -> Terminator2/1
  ISA Atmosphere Model/2 -> Terminator1/1
  Bus Creator2/1 -> Out1/1
  Bus Selector14/3 -> Unit Delay21/1  "<PhiDeg>"
  Bus Selector14/5 -> Unit Delay19/1  "<ThetaDeg>"
  Unit Delay21/1 -> Bus Creator2/3  "Roll_Euler_Deg"
  Knots to m/s2/1 -> Unit Delay17/1
  ISA Atmosphere Model/4 -> Bus Creator2/12  "airDensity_kgm"
  Gain4/1 -> Bus Creator2/2  "V_mps_raw"
  Gain5/1 -> Bus Creator2/11  "Yaccel_raw"
  Bus Selector14/10 -> Unit Delay22/1  "<REFSI_FD_OUT_PIC_dynPres_Pa>"
  [AoA] -> Scope4/2
  Bus Selector14/11 -> Unit Delay16/1  "<NyG>"
  Bus Selector14/13 -> Terminator/1  "<NxG>"
  In1/1 -> Bus Selector14/1
  Bus Selector14/18 -> Knots to m/s3/1  "<CASKts>"
  Gain6/1 -> Bus Creator2/9  "Zaccel_raw"
  Bus Selector14/2 -> Knots to m/s2/1  "<TASKts>"
  Unit Delay/1 -> ft to m/1
  Bus Selector14/12 -> Scope4/1  "<AlphaDeg>"
  Unit Delay15/1 -> Bus Creator2/8  "YawRate_Body_raw"
  Unit Delay19/1 -> Bus Creator2/5  "Pitch_Euler_Deg"
  Bus Selector14/17 -> Unit Delay/1  "<PresAltFt>"
  Bus Selector14/8 -> Unit Delay15/1  "<RDps>"
  Unit Delay20/1 -> Bus Creator2/6  "PitchRate_Body_raw"
  Unit Delay18/1 -> Gain6/1  "NzG_raw (g)"
  Change Direction1/1 -> Ft to m1/1
  Unit Delay2/1 -> Terminator14/1  "CAS_mps"
  ft to m/1 -> ISA Atmosphere Model/1  "Alt_m"
  Unit Delay14/1 -> Bus Creator2/7  "Yaw_Euler_Deg"
  Bus Selector14/1 -> Change Direction1/1  "<VEarthFtps_2>"
  Bus Selector14/9 -> Unit Delay18/1  "<NzG>"
  Bus Selector14/4 -> Unit Delay23/1  "<PDps>"
  Unit Delay17/1 -> Gain4/1  "Sim.TAS"
  Bus Selector14/7 -> Unit Delay14/1  "<PsiDeg>"
  Bus Selector14/6 -> Unit Delay20/1  "<QDps>"
  Unit Delay16/1 -> Gain5/1  "yAccel_Body_mps2_raw"
  Unit Delay22/1 -> Bus Creator2/10  "DynamicPressure_Pa_raw"
  ISA Atmosphere Model/1 -> Terminator16/1  "OAT_K"
  Unit Delay23/1 -> Bus Creator2/4  "RollRate_Body_raw"
  Ft to m1/1 -> Bus Creator2/1  "hdot_m_raw"
  Knots to m/s3/1 -> Unit Delay2/1

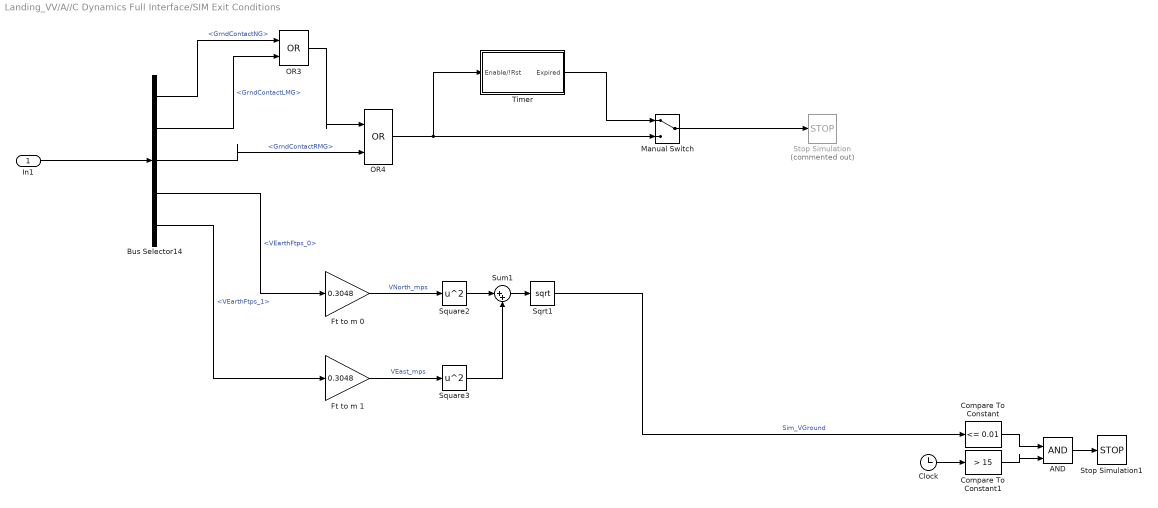
== system Landing_VV/A//C Dynamics Full Interface/SIM Exit Conditions ==
  In1 : Inport
  AND : Logic  IconShape=distinctive  AllPortsSameDT=off  OutDataTypeStr=boolean
  Bus Selector14 : BusSelector  OutputSignals=GrndContactNG,GrndContactLMG,GrndContactRMG,VEarthFtps_0,VEarthFtps_1
  Clock : Clock
  Compare To Constant : simulink/Logic and Bit Operations/Compare To Constant  relop=<=  const=0.01  OutDataTypeStr=boolean
  Compare To Constant1 : simulink/Logic and Bit Operations/Compare To Constant  relop=>  const=15  OutDataTypeStr=boolean
  Ft to m 0 : Gain  Gain=0.3048
  Ft to m 1 : Gain  Gain=0.3048
  Manual Switch : ManualSwitch
  OR3 : Logic  Operator=OR  IconShape=distinctive  AllPortsSameDT=off  OutDataTypeStr=boolean
  OR4 : Logic  Operator=OR  IconShape=distinctive  AllPortsSameDT=off  OutDataTypeStr=boolean
  Sqrt1 : Sqrt  OutputSignalType=real  SaturateOnIntegerOverflow=on
  Square2 : Math  Operator=square  OutputSignalType=real  SaturateOnIntegerOverflow=on
  Square3 : Math  Operator=square  OutputSignalType=real  SaturateOnIntegerOverflow=on
  Stop Simulation : Stop  Commented=on
  Stop Simulation1 : Stop
  Sum1 : Sum  Inputs=|++
  Timer : Subsystem  mask{period=10}
      mask prompts: period "Period [s]"
  wires:
  Bus Selector14/4 -> Ft to m 0/1  "<VEarthFtps_0>"
  Bus Selector14/5 -> Ft to m 1/1  "<VEarthFtps_1>"
  Sum1/1 -> Sqrt1/1
  Square2/1 -> Sum1/1
  Square3/1 -> Sum1/2
  Ft to m 1/1 -> Square3/1  "VEast_mps"
  Ft to m 0/1 -> Square2/1  "VNorth_mps"
  Clock/1 -> Compare To Constant1/1
  Sqrt1/1 -> Compare To Constant/1  "Sim_VGround"
  Compare To Constant1/1 -> AND/2
  Compare To Constant/1 -> AND/1
  AND/1 -> Stop Simulation1/1
  Manual Switch/1 -> Stop Simulation/1
  Bus Selector14/1 -> OR3/1  "<GrndContactNG>"
  In1/1 -> Bus Selector14/1
  Bus Selector14/2 -> OR3/2  "<GrndContactLMG>"
  OR4/1 -> Manual Switch/2, Timer/1(Enable/!Rst)
  Bus Selector14/3 -> OR4/2  "<GrndContactRMG>"
  OR3/1 -> OR4/1
  Timer/1(Expired) -> Manual Switch/1

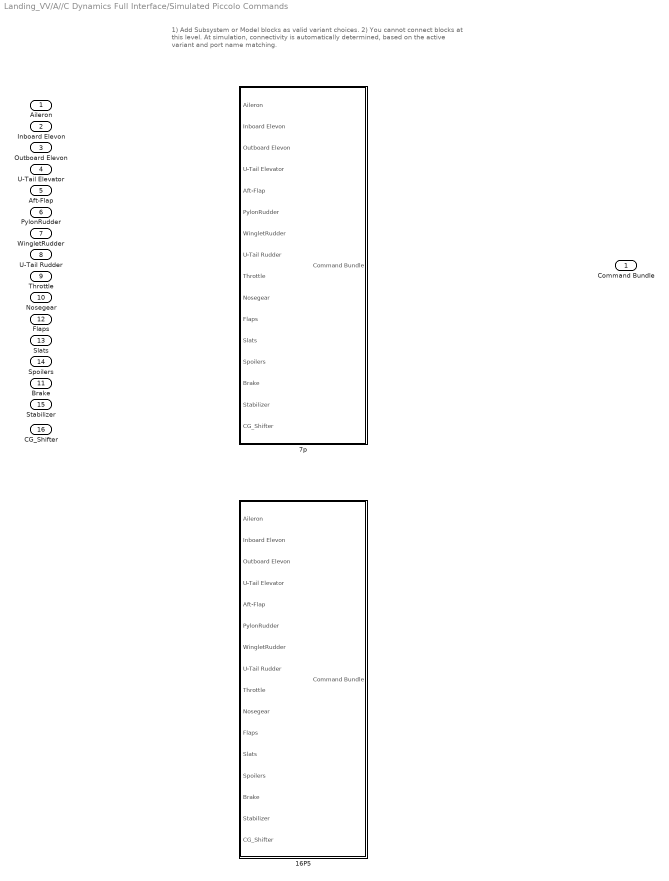
== system Landing_VV/A//C Dynamics Full Interface/Simulated Piccolo Commands ==
  note: 1) Add Subsystem or Model blocks as valid variant choices.
      | 2) You cannot connect blocks at this level. At simulation, connectivity is automatically
      | determined, based on the active variant and port name matching.
  Aileron : Inport
  Inboard Elevon : Inport  Port=2
  Outboard Elevon : Inport  Port=3
  U-Tail Elevator : Inport  Port=4
  Aft-Flap : Inport  Port=5
  "PylonRudder " : Inport  Port=6
  WingletRudder : Inport  Port=7
  U-Tail Rudder : Inport  Port=8
  "Throttle " : Inport  Port=9
  Nosegear : Inport  Port=10
  Brake : Inport  Port=11
  Flaps : Inport  Port=12
  Slats : Inport  Port=13
  Spoilers : Inport  Port=14
  Stabilizer : Inport  Port=15
  CG_Shifter : Inport  Port=16
  16P5 : Subsystem  VariantControl=FTV == 4 && FDMRelease >=38
  7p : Subsystem  VariantControl=FTV == 3 || FDMRelease < 38
  Command Bundle : Outport

== system Landing_VV/A//C Dynamics Full Interface/DLLSimulation/Bus2Vect2 ==
  In1 : Inport
  BusSelector : BusSelector  OutputSignals=REFSI_FD_IN_nmodeRudLhWingCmd_Deg (signal 1),REFSI_FD_IN_nmodeAilLhLowerCmd_Deg (signal 2),REFSI_FD_IN_nmodeAilLhUpperCmd_Deg (signal 3),REFSI_FD_IN_nmodeElvLhOutbdCmd_Deg (signal 4),REFSI_FD_IN_nmodeElvLhInbdCmd_Deg (signal 5),REFSI_FD_IN_nmodeRudLhPylonCmd_Deg (signal 6),REFSI_FD_IN_nmodeRudLhUTailCmd_Deg (signal 7),REFSI_FD_IN_nmodeElvLhUTailCmd_Deg (signal 8),REFSI_FD_IN_nmodeAftFlapCmd_Deg (signal 9),REFSI_FD_IN_nmodeElvRhUTailCmd_Deg (signal 10),REFSI_FD_IN_nmodeRudRhUTailCmd_Deg (signal 11),REFSI_FD_IN_nmodeRudRhPylonCmd_Deg (signal 12),REFSI_FD_IN_nmodeElvRhInbdCmd_Deg (signal 13),REFSI_FD_IN_nmodeElvRhOutbdCmd_Deg (signal 14),REFSI_FD_IN_nmodeAilRhUpperCmd_Deg (signal 15),REFSI_FD_IN_nmodeAilRhLowerCmd_Deg (signal 16),REFSI_FD_IN_nmodeRudRhWingCmd_Deg (signal 17),REFSI_FD_IN_nmodeStabCmd (signal 18),REFSI_FD_IN_nmodeFlapLhOBPosn_Deg (signal 19),REFSI_FD_IN_nmodeFlapLhIBPosn_Deg (signal 20),REFSI_FD_IN_nmodeSlatLhPosn_Deg (signal 21),REFSI_FD_IN_nmodeSlatRhPosn_Deg (signal 22),REFSI_FD_IN_nmodeFlapRhOBPosn_Deg (signal 23),REFSI_FD_IN_nmodeFlapRhIBPosn_Deg (signal 24),REFSI_FD_IN_nmodeTlaLhCmd_Deg (signal 25),REFSI_FD_IN_nmodeTlaLhCmd_Deg (signal 26),EngineLhFuelCut (signal 27),EngineRhFuelCut (signal 28),REFSI_FD_IN_nmodeBrakeCmd (signal 29),REFSI_FD_IN_nmodeNoseGearCmd_Deg (signal 30),REFSI_FD_IN_nmodeSplrLhOutbdCmd_Deg (signal 31),REFSI_FD_IN_nmodeSplrLhInbdCmd_Deg (signal 32),REFSI_FD_IN_nmodeSplrRhInbdCmd_Deg (signal 33),REFSI_FD_IN_nmodeSplrRhOutbdCmd_Deg (signal 34),REFSI_FD_IN_nmodeCgShifterCmd_Ft (signal 35),piccoloInCmd (signal 36),pilotNzCmd_g (signal 37),isControlSurfaceCmdFromSystem (signal 38),nmodeReset (signal 39)
  Mux : Mux  Inputs=39
  Out1 : Outport
  wires:
  Mux/1 -> Out1/1
  In1/1 -> BusSelector/1
